simulink library "Sensors_Block"  (Simulink 8.8)
settings: Solver=VariableStepAuto  StartTime=0.0  StopTime=10.0  RelTol=1e-3
undefined symbols (not defined in the file): CRM
libraries: lib_Sim_CRM x1
settings Model: Creator=cava_da  LastModifiedBy=cava_da

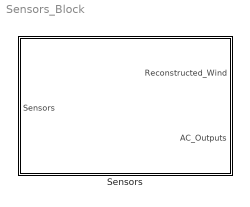
== system Sensors_Block ==
  Sensors : Subsystem

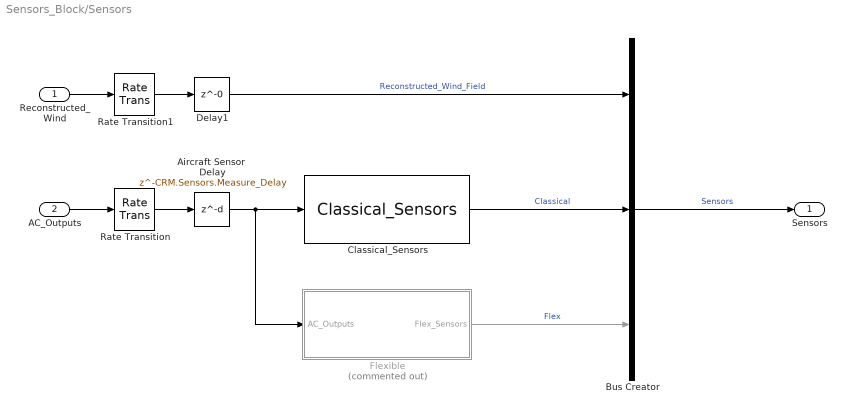
== system Sensors_Block/Sensors ==
  Reconstructed_Wind : Inport
  AC_Outputs : Inport  Port=2
  Aircraft Sensor  Delay : Delay  DelayLength=CRM.Sensors.Measure_Delay
  Bus Creator : BusCreator  Inputs=3
  Classical_Sensors : lib_Sim_CRM/Classical_Sensors  SystemSampleTime=-1
  Delay1 : Delay  DelayLength=0
  Flexible : Subsystem  Commented=on
  Rate Transition : RateTransition  OutPortSampleTime=CRM.FCS.SampleTime
  Rate Transition1 : RateTransition  OutPortSampleTime=CRM.FCS.SampleTime
  Sensors : Outport
  wires:
  Bus Creator/1 -> Sensors/1  "Sensors"
  AC_Outputs/1 -> Rate Transition/1
  Classical_Sensors/1 -> Bus Creator/2  "Classical"
  Flexible/1(Flex_Sensors) -> Bus Creator/3  "Flex"
  Reconstructed_Wind/1 -> Rate Transition1/1
  Delay1/1 -> Bus Creator/1  "Reconstructed_Wind_Field"
  Aircraft Sensor  Delay/1 -> Classical_Sensors/1, Flexible/1(AC_Outputs)
  Rate Transition1/1 -> Delay1/1
  Rate Transition/1 -> Aircraft Sensor  Delay/1

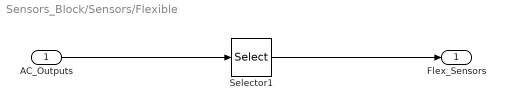
== system Sensors_Block/Sensors/Flexible ==
  AC_Outputs : Inport
  Selector1 : Selector  InputPortWidth=25  IndexOptions=Index vector (dialog)  Indices=[1:25]  OutputSizes=1
  Flex_Sensors : Outport
  wires:
  AC_Outputs/1 -> Selector1/1
  Selector1/1 -> Flex_Sensors/1
